simulink model "EqM"  (R2024b)
settings: Solver=VariableStepAuto  StartTime=0.0  StopTime=10.0  RelTol=1e-3
settings Model: LastModifiedBy=jogos

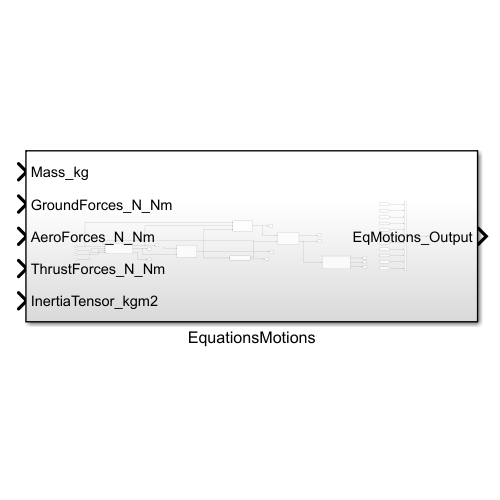
[thumbnail: Simulink's stored preview of the top-level diagram]
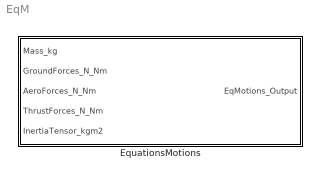
== system EqM ==
  EquationsMotions : Subsystem

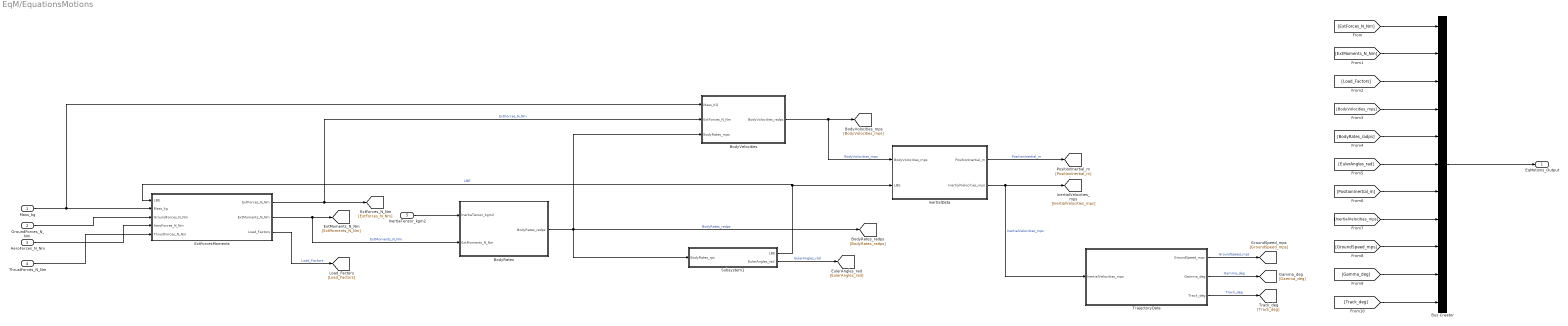
== system EqM/EquationsMotions ==
  Mass_kg : Inport
  GroundForces_N_Nm : Inport  Port=2
  AeroForces_N_Nm : Inport  Port=3
  ThrustForces_N_Nm : Inport  Port=4
  InertiaTensor_kgm2 : Inport  Port=5
  BodyRates : Subsystem
  BodyVelocities : Subsystem
  Bus Creator : BusCreator  Inputs=11
  ExtForcesMoments : Subsystem
  InertialData : Subsystem
  Subsystem1 : Subsystem
  TrajectoryData : Subsystem
  EqMotions_Output : Outport
  wires:
  [Load_Factors] -> Bus Creator/3
  Mass_kg/1 -> BodyVelocities/1(Mass_KG), ExtForcesMoments/2(Mass_kg)
  GroundForces_N_Nm/1 -> ExtForcesMoments/3(GroundForces_N_Nm)
  InertiaTensor_kgm2/1 -> BodyRates/1(InertiaTensor_kgm2)
  [BodyVolocities_mps] -> Bus Creator/4
  ExtForcesMoments/1(ExtForces_N_Nm) -> [ExtForces_N_Nm], BodyVelocities/2(ExtForces_N_Nm)  "ExtForces_N_Nm"
  Subsystem1/1(LBE) -> ExtForcesMoments/1(LBE), InertialData/2(LBE)  "LBE"
  ThrustForces_N_Nm/1 -> ExtForcesMoments/5(ThrustForces_N_Nm)
  [PositionInertial_m] -> Bus Creator/7
  [BodyRates_radps] -> Bus Creator/5
  Bus Creator/1 -> EqMotions_Output/1
  InertialData/1(PositionInertial_m) -> [PositionInertial_m]  "PositionInertial_m"
  BodyRates/1(BodyRates_radps) -> [BodyRates_radps], Subsystem1/1(BodyRates_rps), BodyVelocities/3(BodyRates_mps)  "BodyRates_radps"
  AeroForces_N_Nm/1 -> ExtForcesMoments/4(AeroForces_N_Nm)
  ExtForcesMoments/2(ExtMoments_N_Nm) -> BodyRates/2(ExtMoments_N_Nm), [ExtMoments_N_Nm]  "ExtMoments_N_Nm"
  BodyVelocities/1(BodyVolocities_radps) -> [BodyVolocities_mps], InertialData/1(BodyVolocities_mps)  "BodyVolocities_mps"
  [ExtMoments_N_Nm] -> Bus Creator/2
  InertialData/2(InertialVelocities_mps) -> TrajectoryData/1(InertialVelocities_mps), [InertialVelocities_mps]  "InertialVelocities_mps"
  Subsystem1/2(EulerAngles_rad) -> [EulerAngles_rad]  "EulerAngles_rad"
  ExtForcesMoments/3(Load_Factors) -> [Load_Factors]  "Load_Factors"
  TrajectoryData/3(Track_deg) -> [Track_deg]  "Track_deg"
  [ExtForces_N_Nm] -> Bus Creator/1
  TrajectoryData/2(Gamma_deg) -> [Gamma_deg]  "Gamma_deg"
  [Gamma_deg] -> Bus Creator/10
  TrajectoryData/1(GroundSpeed_mps) -> [GroundSpeed_mps]  "GroundSpeed_mps"
  [EulerAngles_rad] -> Bus Creator/6
  [GroundSpeed_mps] -> Bus Creator/9
  [InertialVelocities_mps] -> Bus Creator/8
  [Track_deg] -> Bus Creator/11

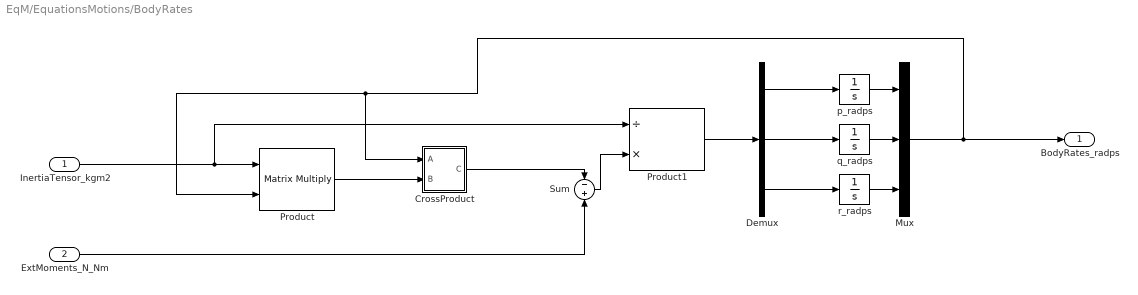
== system EqM/EquationsMotions/BodyRates ==
  InertiaTensor_kgm2 : Inport
  ExtMoments_N_Nm : Inport  Port=2
  CrossProduct : Subsystem
  Demux : Demux  Outputs=3
  Mux : Mux  Inputs=3
  Product : Product  Multiplication=Matrix(*)
  Product1 : Product  Inputs=/*
  Sum : Sum  Inputs=-+
  p_radps : Integrator
  q_radps : Integrator
  r_radps : Integrator
  BodyRates_radps : Outport
  wires:
  r_radps/1 -> Mux/3
  Demux/2 -> q_radps/1
  Product1/1 -> Demux/1
  Demux/3 -> r_radps/1
  q_radps/1 -> Mux/2
  Demux/1 -> p_radps/1
  Sum/1 -> Product1/2
  Product/1 -> CrossProduct/2(B)
  InertiaTensor_kgm2/1 -> Product1/1, Product/1
  CrossProduct/1(C) -> Sum/1
  p_radps/1 -> Mux/1
  ExtMoments_N_Nm/1 -> Sum/2
  Mux/1 -> BodyRates_radps/1, Product/2, CrossProduct/1(A)

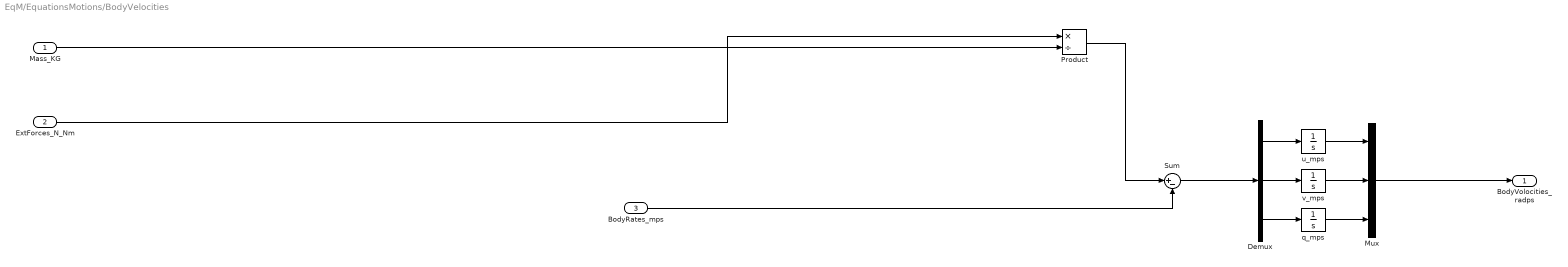
== system EqM/EquationsMotions/BodyVelocities ==
  Mass_KG : Inport
  ExtForces_N_Nm : Inport  Port=2
  BodyRates_mps : Inport  Port=3
  Demux : Demux  Outputs=3
  Mux : Mux  Inputs=3
  Product : Product  Inputs=*/
  Sum : Sum  Inputs=|+-
  q_mps : Integrator
  u_mps : Integrator
  v_mps : Integrator
  BodyVolocities_radps : Outport
  wires:
  q_mps/1 -> Mux/3
  Mux/1 -> BodyVolocities_radps/1
  Demux/1 -> u_mps/1
  Demux/3 -> q_mps/1
  u_mps/1 -> Mux/1
  Demux/2 -> v_mps/1
  Mass_KG/1 -> Product/2
  Product/1 -> Sum/1
  v_mps/1 -> Mux/2
  Sum/1 -> Demux/1
  BodyRates_mps/1 -> Sum/2
  ExtForces_N_Nm/1 -> Product/1

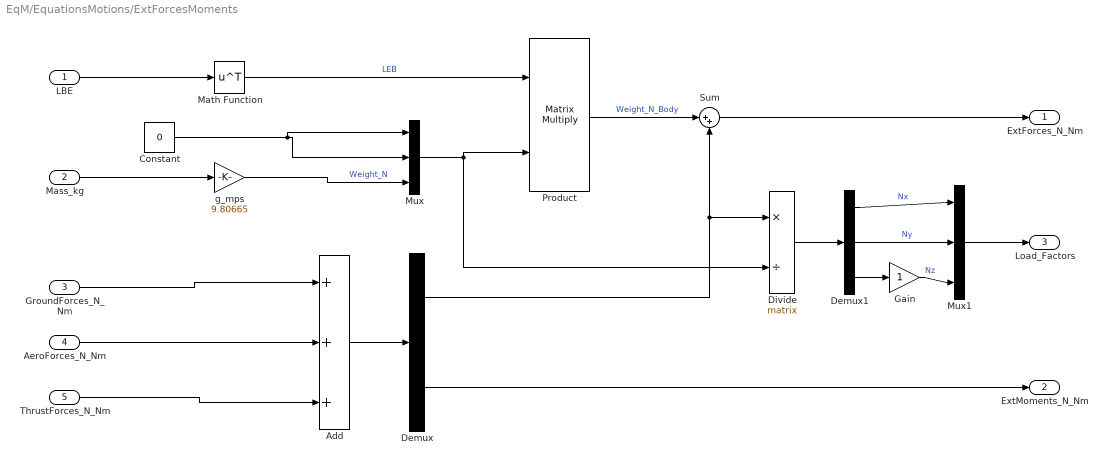
== system EqM/EquationsMotions/ExtForcesMoments ==
  LBE : Inport
  Mass_kg : Inport  Port=2
  GroundForces_N_Nm : Inport  Port=3
  AeroForces_N_Nm : Inport  Port=4
  ThrustForces_N_Nm : Inport  Port=5
  Add : Sum  Inputs=+++
  Constant : Constant  Value=0
  Demux : Demux  Outputs=2
  Demux1 : Demux  Outputs=3
  Divide : Product  Inputs=*/  Multiplication=Matrix(*)
  Gain : Gain
  Math Function : Math  Operator=transpose
  Mux : Mux  Inputs=3
  Mux1 : Mux  Inputs=3
  Product : Product  Multiplication=Matrix(*)
  Sum : Sum  Inputs=|++
  g_mps : Gain  Gain=9.80665
  ExtForces_N_Nm : Outport
  ExtMoments_N_Nm : Outport  Port=2
  Load_Factors : Outport  Port=3
  wires:
  Product/1 -> Sum/1  "Weight_N_Body"
  Mux1/1 -> Load_Factors/1
  Demux1/1 -> Mux1/1  "Nx"
  Demux/2 -> ExtMoments_N_Nm/1
  GroundForces_N_Nm/1 -> Add/1
  Divide/1 -> Demux1/1
  Add/1 -> Demux/1
  Constant/1 -> Mux/2, Mux/1
  Demux/1 -> Sum/2, Divide/1
  LBE/1 -> Math Function/1
  Sum/1 -> ExtForces_N_Nm/1
  ThrustForces_N_Nm/1 -> Add/3
  Mass_kg/1 -> g_mps/1
  Gain/1 -> Mux1/3  "Nz"
  Mux/1 -> Product/2, Divide/2
  Math Function/1 -> Product/1  "LEB"
  g_mps/1 -> Mux/3  "Weight_N"
  AeroForces_N_Nm/1 -> Add/2
  Demux1/3 -> Gain/1
  Demux1/2 -> Mux1/2  "Ny"

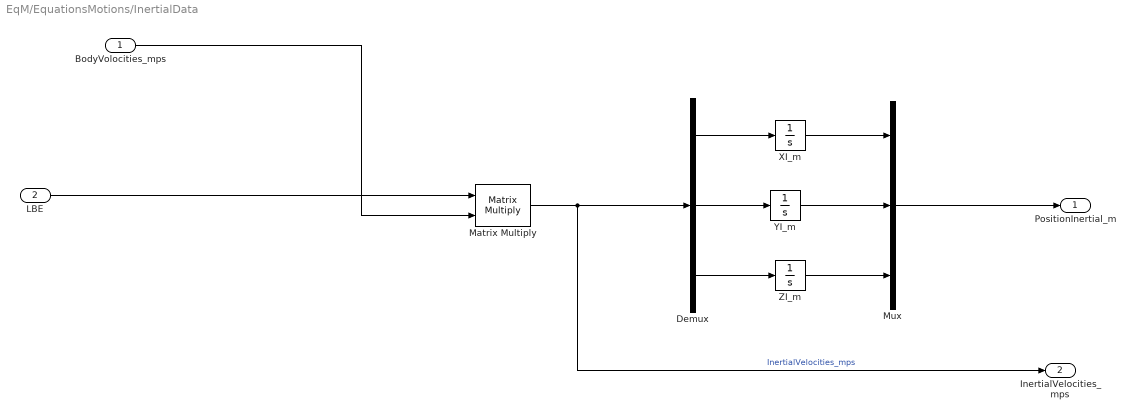
== system EqM/EquationsMotions/InertialData ==
  BodyVolocities_mps : Inport
  LBE : Inport  Port=2
  Demux : Demux  Outputs=3
  Matrix Multiply : Product  Multiplication=Matrix(*)
  Mux : Mux  Inputs=3
  XI_m : Integrator
  YI_m : Integrator
  ZI_m : Integrator
  PositionInertial_m : Outport
  InertialVelocities_mps : Outport  Port=2
  wires:
  XI_m/1 -> Mux/1
  Demux/3 -> ZI_m/1
  Demux/1 -> XI_m/1
  Matrix Multiply/1 -> InertialVelocities_mps/1, Demux/1  "InertialVelocities_mps"
  ZI_m/1 -> Mux/3
  YI_m/1 -> Mux/2
  Demux/2 -> YI_m/1
  BodyVolocities_mps/1 -> Matrix Multiply/2
  LBE/1 -> Matrix Multiply/1
  Mux/1 -> PositionInertial_m/1

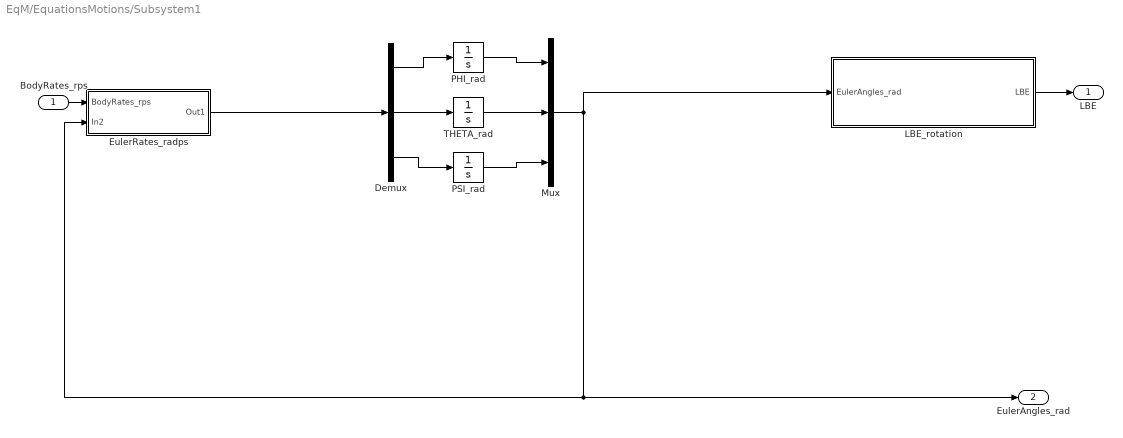
== system EqM/EquationsMotions/Subsystem1 ==
  BodyRates_rps : Inport
  Demux : Demux  Outputs=3
  EulerRates_radps : Subsystem
  LBE_rotation : Subsystem
  Mux : Mux  Inputs=3
  PHI_rad : Integrator
  PSI_rad : Integrator
  THETA_rad : Integrator
  LBE : Outport
  EulerAngles_rad : Outport  Port=2
  wires:
  Demux/2 -> THETA_rad/1
  PSI_rad/1 -> Mux/3
  PHI_rad/1 -> Mux/1
  THETA_rad/1 -> Mux/2
  Demux/1 -> PHI_rad/1
  Demux/3 -> PSI_rad/1
  LBE_rotation/1(LBE) -> LBE/1
  BodyRates_rps/1 -> EulerRates_radps/1(BodyRates_rps)
  EulerRates_radps/1(Out1) -> Demux/1
  Mux/1 -> EulerRates_radps/2(In2), EulerAngles_rad/1, LBE_rotation/1(EulerAngles_rad)

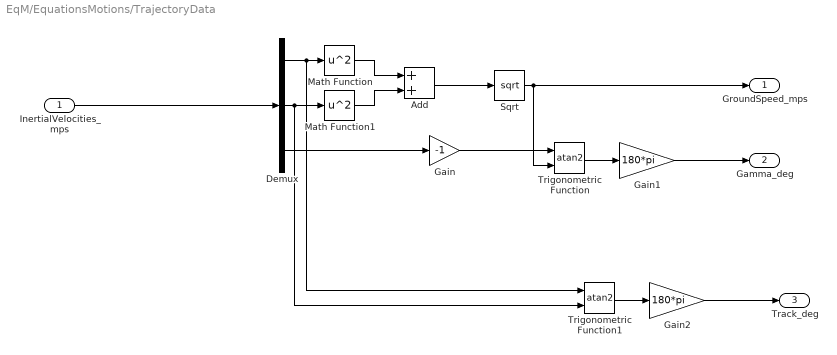
== system EqM/EquationsMotions/TrajectoryData ==
  InertialVelocities_mps : Inport
  Add : Sum
  Demux : Demux  Outputs=3
  Gain : Gain  Gain=-1
  Gain1 : Gain  Gain=180*pi
  Gain2 : Gain  Gain=180*pi
  Math Function : Math  Operator=square
  Math Function1 : Math  Operator=square
  Sqrt : Sqrt
  Trigonometric Function : Trigonometry  Operator=atan2
  Trigonometric Function1 : Trigonometry  Operator=atan2
  GroundSpeed_mps : Outport
  Gamma_deg : Outport  Port=2
  Track_deg : Outport  Port=3
  wires:
  Add/1 -> Sqrt/1
  Sqrt/1 -> GroundSpeed_mps/1, Trigonometric Function/2
  Demux/3 -> Gain/1
  Trigonometric Function1/1 -> Gain2/1
  Math Function/1 -> Add/1
  Gain/1 -> Trigonometric Function/1
  Gain2/1 -> Track_deg/1
  Demux/1 -> Trigonometric Function1/1, Math Function/1
  Demux/2 -> Trigonometric Function1/2, Math Function1/1
  Gain1/1 -> Gamma_deg/1
  Math Function1/1 -> Add/2
  Trigonometric Function/1 -> Gain1/1
  InertialVelocities_mps/1 -> Demux/1

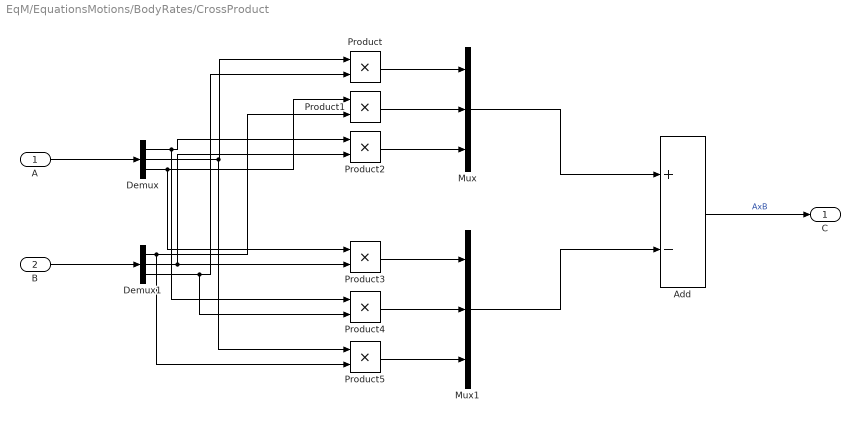
== system EqM/EquationsMotions/BodyRates/CrossProduct ==
  A : Inport
  B : Inport  Port=2
  Add : Sum  Inputs=+-
  Demux : Demux  Outputs=3
  Demux1 : Demux  Outputs=3
  Mux : Mux  Inputs=3
  Mux1 : Mux  Inputs=3
  Product{,1..5} (6 alike) : Product
  C : Outport
  wires:
  Product5/1 -> Mux1/3
  B/1 -> Demux1/1
  A/1 -> Demux/1
  Product/1 -> Mux/1
  Demux/2 -> Product5/1, Product/1
  Product4/1 -> Mux1/2
  Mux/1 -> Add/1
  Demux/1 -> Product4/1, Product2/1
  Demux/3 -> Product3/1, Product1/1
  Product1/1 -> Mux/2
  Product2/1 -> Mux/3
  Product3/1 -> Mux1/1
  Demux1/3 -> Product4/2, Product/2
  Demux1/1 -> Product5/2, Product1/2
  Add/1 -> C/1  "AxB"
  Mux1/1 -> Add/2
  Demux1/2 -> Product3/2, Product2/2

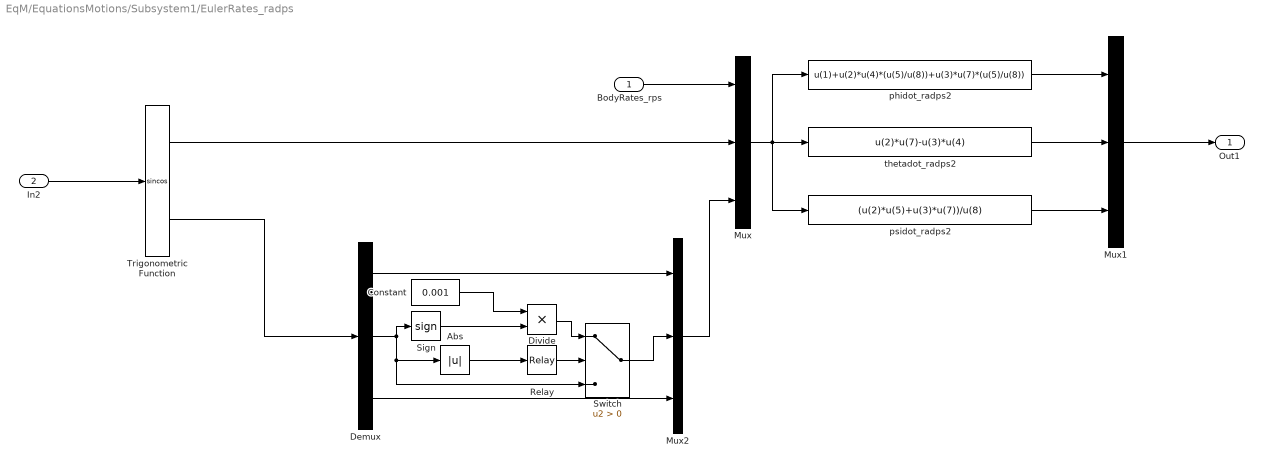
== system EqM/EquationsMotions/Subsystem1/EulerRates_radps ==
  BodyRates_rps : Inport
  In2 : Inport  Port=2
  Abs : Abs  SaturateOnIntegerOverflow=off
  Constant : Constant  Value=0.001
  Demux : Demux  Outputs=3
  Divide : Product  Inputs=**
  Mux : Mux  Inputs=3
  Mux1 : Mux  Inputs=3
  Mux2 : Mux  Inputs=3
  Relay : Relay  OnSwitchValue=0.001  OffSwitchValue=0  OnOutputValue=0  OffOutputValue=1
  Sign : Signum
  Switch : Switch  Criteria=u2 > Threshold  SaturateOnIntegerOverflow=off  InputSameDT=off
  Trigonometric Function : Trigonometry  Operator=sincos
  phidot_radps2 : Fcn  Expr=u(1)+u(2)*u(4)*(u(5)/u(8))+u(3)*u(7)*(u(5)/u(8))
  psidot_radps2 : Fcn  Expr=(u(2)*u(5)+u(3)*u(7))/u(8)
  thetadot_radps2 : Fcn  Expr=u(2)*u(7)-u(3)*u(4)
  Out1 : Outport
  wires:
  Divide/1 -> Switch/1
  Demux/3 -> Mux2/3
  BodyRates_rps/1 -> Mux/1
  Demux/1 -> Mux2/1
  Trigonometric Function/1 -> Mux/2
  In2/1 -> Trigonometric Function/1
  Mux1/1 -> Out1/1
  Constant/1 -> Divide/1
  Sign/1 -> Divide/2
  Switch/1 -> Mux2/2
  Demux/2 -> Switch/3, Abs/1, Sign/1
  phidot_radps2/1 -> Mux1/1
  Mux/1 -> phidot_radps2/1, thetadot_radps2/1, psidot_radps2/1
  thetadot_radps2/1 -> Mux1/2
  Mux2/1 -> Mux/3
  Relay/1 -> Switch/2
  Trigonometric Function/2 -> Demux/1
  Abs/1 -> Relay/1
  psidot_radps2/1 -> Mux1/3

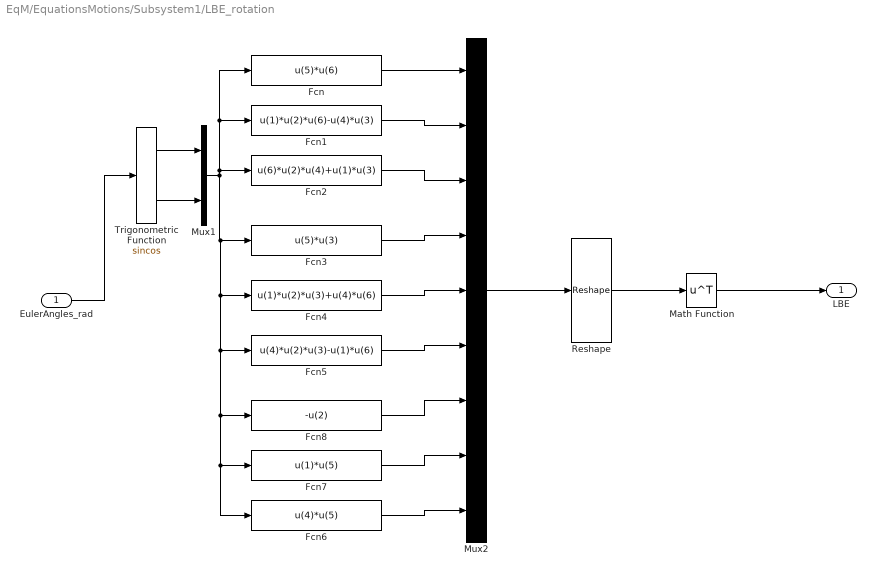
== system EqM/EquationsMotions/Subsystem1/LBE_rotation ==
  EulerAngles_rad : Inport
  Fcn : Fcn  Expr=u(5)*u(6)
  Fcn1 : Fcn  Expr=u(1)*u(2)*u(6)-u(4)*u(3)
  Fcn2 : Fcn  Expr=u(6)*u(2)*u(4)+u(1)*u(3)
  Fcn3 : Fcn  Expr=u(5)*u(3)
  Fcn4 : Fcn  Expr=u(1)*u(2)*u(3)+u(4)*u(6)
  Fcn5 : Fcn  Expr=u(4)*u(2)*u(3)-u(1)*u(6)
  Fcn6 : Fcn  Expr=u(4)*u(5)
  Fcn7 : Fcn  Expr=u(1)*u(5)
  Fcn8 : Fcn  Expr=-u(2)
  Math Function : Math  Operator=transpose
  Mux1 : Mux  Inputs=2
  Mux2 : Mux  Inputs=9
  Reshape : Reshape  OutputDimensionality=Customize  OutputDimensions=[3,1]
  Trigonometric Function : Trigonometry  Operator=sincos
  LBE : Outport
  wires:
  Fcn6/1 -> Mux2/9
  Fcn2/1 -> Mux2/3
  Fcn3/1 -> Mux2/4
  Trigonometric Function/2 -> Mux1/2
  Mux1/1 -> Fcn6/1, Fcn7/1, Fcn8/1, Fcn5/1, Fcn4/1, Fcn3/1, Fcn2/1, Fcn1/1, Fcn/1
  Fcn4/1 -> Mux2/5
  Math Function/1 -> LBE/1
  Fcn/1 -> Mux2/1
  Fcn7/1 -> Mux2/8
  EulerAngles_rad/1 -> Trigonometric Function/1
  Reshape/1 -> Math Function/1
  Fcn5/1 -> Mux2/6
  Fcn8/1 -> Mux2/7
  Fcn1/1 -> Mux2/2
  Trigonometric Function/1 -> Mux1/1
  Mux2/1 -> Reshape/1
